simulink model "FYPPP"  (R2021b)
settings: Solver=VariableStepAuto  StartTime=0.0  StopTime=7200  MaxStep=10  RelTol=1e-3  EnableMultiTasking=on
PreLoadFcn:
  | ssc_lithium_cell_1RC_ini
undefined symbols (not defined in the file): Battery, C1, Capacity, DiscIntNeverNeededParam, Em, Ion, Lithium, Qe_init, R0, R1
libraries: fl_lib x50, nesl_utility x17, LiBatteryElements_lib x12, fl_ps_legacy_lib x9, spsBatteryLib x4, spsSeriesRLCBranchLib x4, spsIGBTLib x3, ee_lib x2, spsIdealSwitchLib x2, spsBreakerLib x2, spspowerguiLib x2, spsDCVoltageSourceLib x1
(part 1 of 2)
CloseFcn:
  | try,close(h1_ssc_lithium_battery_with_fault),end
  | clear h1_ssc_lithium_battery_with_fault
  | 
  | clear simlog_ssc_lithium_battery_with_fault
Description:
  | Lithium-Ion Battery Pack With Fault
  | 
  | Copyright 2008-2017 The MathWorks, Inc.
settings Model: Creator=MathWorks  LastModifiedBy=91875
settings SolverCC: AlgebraicLoopSolver=TrustRegion
settings DataIOCC: LimitDataPoints=on  SaveFormat=Array  ReturnWorkspaceOutputs=off
settings OptimizationCC: LifeSpan=inf
settings DebuggingCC: AllowSymbolicDim=off  SFUnexpectedBacktrackingDiag=warning  SFNoUnconditionalDefaultTransitionDiag=warning  SFExecutionAtInitializationDiag=none  SFMachineParentedDataDiag=warning  ArithmeticOperatorsInVariantConditions=warning
settings HardwareCC: ProdBitPerPointer=32  ProdBitPerSizeT=32  ProdBitPerPtrDiffT=32  ProdLargestAtomicFloat=None  ProdIntDivRoundTo=Undefined  ProdEndianess=Unspecified  ProdWordSize=32  ProdHWDeviceType=32-bit Generic
settings ModelReferenceCC: PropagateSignalLabelsOutOfModel=off
settings SFSimCC: SimUseLocalCustomCode=off  CustomCodeUndefinedFunction=UseInterfaceOnly
settings RTWCC: RTWUseLocalCustomCode=off
settings CodeAppCC: StateflowObjectComments=on
settings GRTTargetCC: TargetLangStandard=C89/C90 (ANSI)
settings ConfigComp: CovMetricSettings=dw  CovSaveCumulativeToWorkspaceVar=on  CovSaveSingleToWorkspaceVar=on  CovExternalEMLEnable=off
settings SimscapeCC: SimscapeNormalizeSystem=off  SimscapeLogType=all  SimscapeLogSimulationStatistics=on  SimscapeLogName=simlog_ssc_lithium_battery_with_fault  SimscapeLogDataHistory=10000

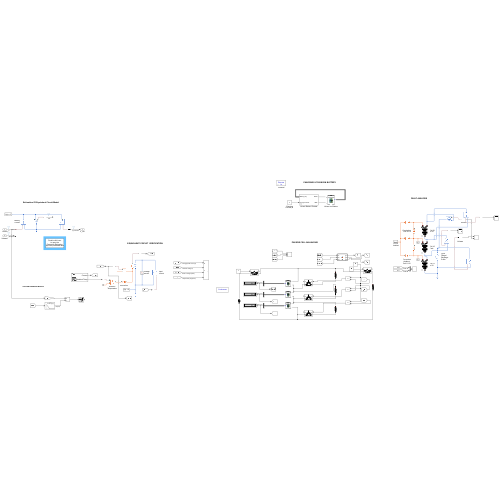
[thumbnail: Simulink's stored preview of the top-level diagram]
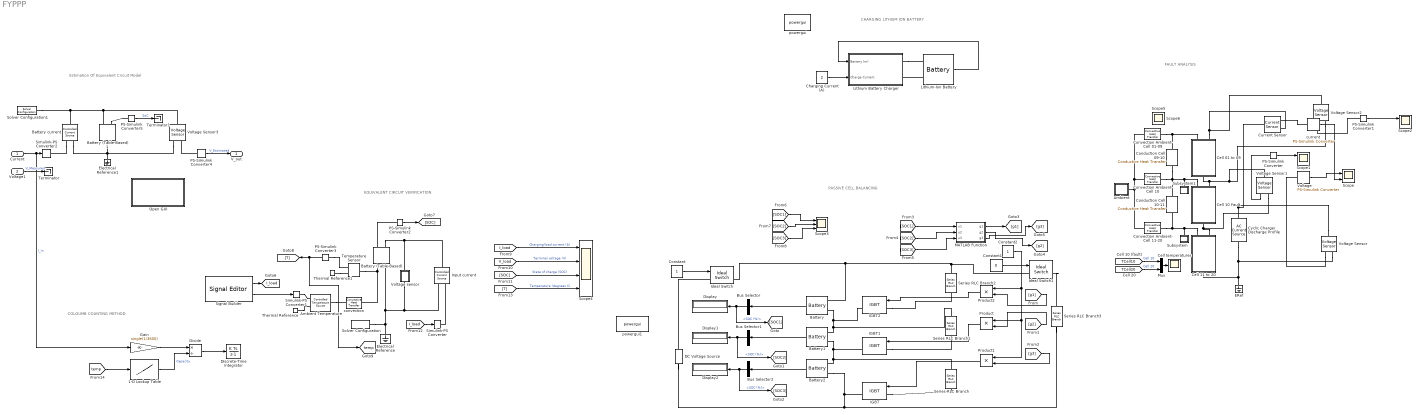
== system FYPPP ==
  note: COLOUMB COUNTING METHOD
  note: Estimation Of Equivalent Circuit Model
  note: EQUIVALENT CIRCUIT VERIFICATION
  note: PASSIVE CELL BALANCING
  note: CHARGING LITHIUM ION BATTERY
  note: FAULT ANALYSIS
  Current : Inport
  Voltage1 : Inport  Port=2
  1-D Lookup Table : Lookup_n-D  NumberOfTableDimensions=1  BreakpointsForDimension1=single(Battery(1).Temperature_LUT)  Table=single(Battery(1).Capacity_LUT)  InternalRulePriority=Speed  RndMeth=Simplest  InputSameDT=on
  Ambient : Subsystem
  Ambient Temperature : fl_lib/Thermal/Thermal Sources/Controlled Temperature Source
  Battery : spsBatteryLib/Battery  BatType=Lithium-Ion  ShowTempParam=off  ThermalPreset=no  ShowAgeParam=off  NomV=3.7  NomQ=5.4  SOC=32  Batt_Tr=30  PresetModel=on  MaxQ=5.4  MinV=2.775  FullV=4.3068  Dis_rate=2.3478  R=0.0068519  Normal_OP=4.8835  expZone="[3.9974      0.2653]"  current=[6.5 13 32.5]  Units=Time  Tci=20  NomT=20  T2=-30  MaxQ2=4.8  FullV2=7.1  Normal_OP2=5.655  expZone2="[6.58           1]"  Rca=0.6  ti=2000  Dp=0  Neq0=0  Tsim=1e6  Ta1=25  Qeol=5.4*0.9  Reol=0.013333*1.2  Char_age=[2.3478, 3]  Dis_age=[2.3478, 10]  N1=1500  N2=10500  N3=1000  N4=1400  Ta2=45  N5=950
  Battery (Table-Based) : ee_lib/Sources/Battery (Table-Based)  SOC_vec=Battery.SOC_LUT  T_dependence=ee.enum.temperature_dependence.yes  prm_dir=ee.enum.battery.prm_dir.noCurrentDirectionality  T_vec=Battery.Temperature_LUT K  V0_mat=Battery.Em_LUT V  V0_vec=[3.1, 3.27, 3.31, 3.5] V  R0_mat=Battery.R0_LUT Ohm  R0_vec=[.015, .017, .012, .013] Ohm  R0_dis_mat=[.03, .015, .002; .04, .017, .008; .039, .012, .006; .027, .013, .021] Ohm  R0_dis_vec=[.015, .017, .012, .013] Ohm  R0_ch_mat=[.03, .015, .002; .04, .017, .008; .039, .012, .006; .027, .013, .021] Ohm  R0_ch_vec=[.015, .017, .012, .013] Ohm  AH_vec=Battery.Capacity_LUT hr*A  AH=4.1 hr*A  prm_leak=1  Rleak_vec=[8000, 7000, 6000] Ohm  Rleak=7e3 Ohm  extrapolation_option=ee.enum.extrapolation.linear  prm_dyn=2  R1_mat=Battery.R1_LUT Ohm  R1_vec=[.076, .022, .007, .043] Ohm  tau1_mat=Battery.R1_LUT.*Battery.C1_LUT s  tau1_vec=[148, 110, 27, 22] s  R2_mat=[.014, .382, .407; .028, .006, .007; .014, .007, .006; .333, .956, .912] Ohm  R2_vec=[.382, .006, .007, .956] Ohm  tau2_mat=[1, 44, 5644; 11, 24, 506; 2, 14, 330; 3310, 13419, 30216] s  tau2_vec=[44, 24, 14, 13419] s  R3_mat=[.014, .382, .407; .028, .006, .007; .014, .007, .006; .333, .956, .912] Ohm  R3_vec=[.382, .006, .007, .956] Ohm  tau3_mat=[1, 44, 5644; 11, 24, 506; 2, 14, 330; 3310, 13419, 30216] s  tau3_vec=[44, 24, 14, 13419] s  R4_mat=[.014, .382, .407; .028, .006, .007; .014, .007, .006; .333, .956, .912] Ohm  R4_vec=[.382, .006, .007, .956] Ohm  tau4_mat=[1, 44, 5644; 11, 24, 506; 2, 14, 330; 3310, 13419, 30216] s  tau4_vec=[44, 24, 14, 13419] s  R5_mat=[.014, .382, .407; .028, .006, .007; .014, .007, .006; .333, .956, .912] Ohm  R5_vec=[.382, .006, .007, .956] Ohm  tau5_mat=[1, 44, 5644; 11, 24, 506; 2, 14, 330; 3310, 13419, 30216] s  tau5_vec=[44, 24, 14, 13419] s  prm_fade=ee.enum.battery.prm_fade.equations  N0=100  dV0=0  dR0=0  dAH=0  dRleak=0  dR1=0  dR2=0  dR3=0  dR4=0  dR5=0  N0vec=[100, 200, 300]  Tfadevec=[298.15, 323.15] K  dV0vec=[0, 0, 0]  dR0vec=[0, 0, 0]  dAHvec=[0, 0, 0]  dRleakvec=[0, 0, 0]  dR1vec=[0, 0, 0]  dR2vec=[0, 0, 0]  dR3vec=[0, 0, 0]  dR4vec=[0, 0, 0]  dR5vec=[0, 0, 0]  dV0mat=[0, 0; 0, 0; 0, 0]  dR0mat=[0, 0; 0, 0; 0, 0]  dAHmat=[0, 0; 0, 0; 0, 0]  dRleakmat=[0, 0; 0, 0; 0, 0]  dR1mat=[0, 0; 0, 0; 0, 0]  dR2mat=[0, 0; 0, 0; 0, 0]  dR3mat=[0, 0; 0, 0; 0, 0]  dR4mat=[0, 0; 0, 0; 0, 0]  dR5mat=[0, 0; 0, 0; 0, 0]  prm_age=ee.enum.battery.prm_age.disabled  prm_age_OCV=ee.enum.battery.prm_age_OCV.OCV  OCV_age=0.9  SOC_age=0.6  storage_dt_age_vec=[0] d  storage_T_age_vec=[273] K  OCV_scaling_age=2.2134e6  OCV_offset_age=1.632e6  temp_exp_age=0.515833569 V  t_exp_age=0.75  T_age_vec=[273.15, 298.15, 323.15] K  dt_age_vec=[90, 180, 270, 360] d  dR0_age_vec=[0, 0, 0]  t_meas_dR0_age=100 d  dR0_age_mat=[0, 0, 0; 0, 0, 0; 0, 0, 0; 0, 0, 0]  temperature=Battery.T_init K  i_specify=off  i_priority=None  i=0 A  i_nominal_specify=off  i_nominal_unit=A  i_nominal_value=1  v_specify=off  v_priority=None  v=0 V  v_nominal_specify=off  v_nominal_unit=V  v_nominal_value=1  stateOfCharge_specify=on  stateOfCharge_priority=High  stateOfCharge=(Battery.Capacity_LUT(2) - Battery.Qe_init)/Battery.Capacity_LUT(2)  stateOfCharge_nominal_specify=off  stateOfCharge_nominal_unit=1  stateOfCharge_nominal_value=1  num_cycles_specify=off  num_cycles_priority=High  num_cycles=0  num_cycles_nominal_specify=off  num_cycles_nominal_unit=1  num_cycles_nominal_value=1  thermal_mass=Battery.cell_Cp_heat*Battery.cell_mass J/K  temperature_specify=on  temperature_priority=High  temperature_nominal_specify=off  temperature_nominal_unit=K  temperature_nominal_value=1
      settings: SourceProductBaseCode=PS  InternalSimscapePortConfiguration="{\"Bottom\":[],\"Left\":[{\"id\":\"p\",\"label\":\"+\",\"type\":\"foundation.electrical.electrical\"},{\"id\":\"soc\",\"label\":\"SOC\",\"type\":\"output\"}],\"Right\":[{\"id\":\"n\",\"label\":\"-\",\"type\":\"foundation.electrical.electrical\"},{\"id\":\"H\",\"label\":\"H\",\"type\":\"foundation.thermal.thermal\"}],\"Top\":[]}"
  Battery (Table-Based)1 : ee_lib/Sources/Battery (Table-Based)  SOC_vec=SOC_LUT  T_dependence=ee.enum.temperature_dependence.no  prm_dir=ee.enum.battery.prm_dir.noCurrentDirectionality  T_vec=[273.15, 298.15] K  V0_mat=[Em, Em] V  V0_vec=Em V  R0_mat=[R0, R0] Ohm  R0_vec=R0 Ohm  R0_dis_mat=[.03, .015, .002; .04, .017, .008; .039, .012, .006; .027, .013, .021] Ohm  R0_dis_vec=[.015, .017, .012, .013] Ohm  R0_ch_mat=[.03, .015, .002; .04, .017, .008; .039, .012, .006; .027, .013, .021] Ohm  R0_ch_vec=[.015, .017, .012, .013] Ohm  AH_vec=[Capacity, Capacity] hr*A  AH=Capacity hr*A  prm_leak=ee.enum.battery.prm_leak.disabled  Rleak_vec=[8000, 7000, 6000] Ohm  Rleak=7e3 Ohm  extrapolation_option=ee.enum.extrapolation.linear  prm_dyn=ee.enum.battery.prm_dyn.rc1  R1_mat=[R1, R1] Ohm  R1_vec=R1 Ohm  tau1_mat=[R1.*C1, R1.*C1] s  tau1_vec=R1.*C1 s  R2_mat=[.014, .382, .407; .028, .006, .007; .014, .007, .006; .333, .956, .912] Ohm  R2_vec=[.382, .006, .007, .956] Ohm  tau2_mat=[1, 44, 5644; 11, 24, 506; 2, 14, 330; 3310, 13419, 30216] s  tau2_vec=[44, 24, 14, 13419] s  R3_mat=[.014, .382, .407; .028, .006, .007; .014, .007, .006; .333, .956, .912] Ohm  R3_vec=[.382, .006, .007, .956] Ohm  tau3_mat=[1, 44, 5644; 11, 24, 506; 2, 14, 330; 3310, 13419, 30216] s  tau3_vec=[44, 24, 14, 13419] s  R4_mat=[.014, .382, .407; .028, .006, .007; .014, .007, .006; .333, .956, .912] Ohm  R4_vec=[.382, .006, .007, .956] Ohm  tau4_mat=[1, 44, 5644; 11, 24, 506; 2, 14, 330; 3310, 13419, 30216] s  tau4_vec=[44, 24, 14, 13419] s  R5_mat=[.014, .382, .407; .028, .006, .007; .014, .007, .006; .333, .956, .912] Ohm  R5_vec=[.382, .006, .007, .956] Ohm  tau5_mat=[1, 44, 5644; 11, 24, 506; 2, 14, 330; 3310, 13419, 30216] s  tau5_vec=[44, 24, 14, 13419] s  prm_fade=ee.enum.battery.prm_fade.equations  N0=100  dV0=0  dR0=0  dAH=0  dRleak=0  dR1=0  dR2=0  dR3=0  dR4=0  dR5=0  N0vec=[100, 200, 300]  Tfadevec=[298.15, 323.15] K  dV0vec=[0, 0, 0]  dR0vec=[0, 0, 0]  dAHvec=[0, 0, 0]  dRleakvec=[0, 0, 0]  dR1vec=[0, 0, 0]  dR2vec=[0, 0, 0]  dR3vec=[0, 0, 0]  dR4vec=[0, 0, 0]  dR5vec=[0, 0, 0]  dV0mat=[0, 0; 0, 0; 0, 0]  dR0mat=[0, 0; 0, 0; 0, 0]  dAHmat=[0, 0; 0, 0; 0, 0]  dRleakmat=[0, 0; 0, 0; 0, 0]  dR1mat=[0, 0; 0, 0; 0, 0]  dR2mat=[0, 0; 0, 0; 0, 0]  dR3mat=[0, 0; 0, 0; 0, 0]  dR4mat=[0, 0; 0, 0; 0, 0]  dR5mat=[0, 0; 0, 0; 0, 0]  prm_age=ee.enum.battery.prm_age.disabled  prm_age_OCV=ee.enum.battery.prm_age_OCV.OCV  OCV_age=0.9  SOC_age=0.6  storage_dt_age_vec=[0] d  storage_T_age_vec=[273] K  OCV_scaling_age=2.2134e6  OCV_offset_age=1.632e6  temp_exp_age=0.515833569 V  t_exp_age=0.75  T_age_vec=[273.15, 298.15, 323.15] K  dt_age_vec=[90, 180, 270, 360] d  dR0_age_vec=[0, 0, 0]  t_meas_dR0_age=100 d  dR0_age_mat=[0, 0, 0; 0, 0, 0; 0, 0, 0; 0, 0, 0]  temperature=298.15 K  i_specify=off  i_priority=None  i=0 A  i_nominal_specify=off  i_nominal_unit=A  i_nominal_value=1  v_specify=off  v_priority=None  v=0 V  v_nominal_specify=off  v_nominal_unit=V  v_nominal_value=1  stateOfCharge_specify=off  stateOfCharge_priority=High  stateOfCharge=1  stateOfCharge_nominal_specify=off  stateOfCharge_nominal_unit=1  stateOfCharge_nominal_value=1  num_cycles_specify=off  num_cycles_priority=High  num_cycles=0  num_cycles_nominal_specify=off  num_cycles_nominal_unit=1  num_cycles_nominal_value=1  thermal_mass=30000 J/K  temperature_specify=off  temperature_priority=High  temperature_nominal_specify=off  temperature_nominal_unit=K  temperature_nominal_value=1
      settings: SourceProductBaseCode=PS  InternalSimscapePortConfiguration="{\"Bottom\":[],\"Left\":[{\"id\":\"p\",\"label\":\"+\",\"type\":\"foundation.electrical.electrical\"},{\"id\":\"soc\",\"label\":\"SOC\",\"type\":\"output\"}],\"Right\":[{\"id\":\"n\",\"label\":\"-\",\"type\":\"foundation.electrical.electrical\"}],\"Top\":[]}"
  Battery current : fl_lib/Electrical/Electrical Sources/Controlled Current Source
  Battery1 : spsBatteryLib/Battery  BatType=Lithium-Ion  ShowTempParam=off  ThermalPreset=no  ShowAgeParam=off  NomV=3.7  NomQ=5.4  SOC=28  Batt_Tr=30  PresetModel=on  MaxQ=5.4  MinV=2.775  FullV=4.3068  Dis_rate=2.3478  R=0.0068519  Normal_OP=4.8835  expZone="[3.9974      0.2653]"  current=[6.5 13 32.5]  Units=Time  Tci=20  NomT=20  T2=-30  MaxQ2=4.8  FullV2=7.1  Normal_OP2=5.655  expZone2="[6.58           1]"  Rca=0.6  ti=2000  Dp=0  Neq0=0  Tsim=1e6  Ta1=25  Qeol=5.4*0.9  Reol=0.013333*1.2  Char_age=[2.3478, 3]  Dis_age=[2.3478, 10]  N1=1500  N2=10500  N3=1000  N4=1400  Ta2=45  N5=950
  Battery2 : spsBatteryLib/Battery  BatType=Lithium-Ion  ShowTempParam=off  ThermalPreset=no  ShowAgeParam=off  NomV=3.7  NomQ=5.4  SOC=26  Batt_Tr=30  PresetModel=on  MaxQ=5.4  MinV=2.775  FullV=4.3068  Dis_rate=2.3478  R=0.0068519  Normal_OP=4.8835  expZone="[3.9974      0.2653]"  current=[6.5 13 32.5]  Units=Time  Tci=20  NomT=20  T2=-30  MaxQ2=4.8  FullV2=7.1  Normal_OP2=5.655  expZone2="[6.58           1]"  Rca=0.6  ti=2000  Dp=0  Neq0=0  Tsim=1e6  Ta1=25  Qeol=5.4*0.9  Reol=0.013333*1.2  Char_age=[2.3478, 3]  Dis_age=[2.3478, 10]  N1=1500  N2=10500  N3=1000  N4=1400  Ta2=45  N5=950
  Bus Selector : BusSelector  OutputSignals=SOC (%)
  Bus Selector1 : BusSelector  OutputSignals=SOC (%)
  Bus Selector2 : BusSelector  OutputSignals=SOC (%)
  Cell temperatures : Scope
  Cell 01 to 09 : Subsystem  Tag=PublishSubsystem  mask(Lithium cell (one RC-branch equivalent circuit)){Ncells=9, Qe_init=Qe_init, T_init=Battery.T_init, Capacity_LUT=Battery.Capacity_LUT, Em_LUT=Battery.Em_LUT, R0_LUT=Battery.R0_LUT, R1_LUT=Battery.R1_LUT, C1_LUT=Battery.C1_LUT, cell_mass=Battery.cell_mass, cell_Cp_heat=Battery.cell_Cp_heat, SOC_LUT=Battery.SOC_LUT, Temperature_LUT=Battery.Temperature_LUT}
      mask prompts: Ncells "Number of series-connected cells"; Qe_init "Initial cell charge deficit (A*hr)"; T_init "Initial cell temperature (K)"; Capacity_LUT "Capacity (A*hr, 1xN table)"; Em_LUT "Em open-circuit voltage, Em (volts, MxN table)"; R0_LUT "R0 terminal resistance (ohms, MxN table)"; R1_LUT "R1 cell resistance (ohms, MxN table)"; C1_LUT "C1 capacitance (farads, MxN table)"; cell_mass "Cell mass (kg)"; cell_Cp_heat "Cell specific heat (J/kg/K)"; SOC_LUT "SOC table breakpoints (Mx1 array)"; Temperature_LUT "Temperature table breakpoints (K, 1xN array)"
      mask DialogControl ParameterTabVar0 Prompt: Main
      mask DialogControl ParameterTabVar01 Prompt: Electrical (per cell)
      mask DialogControl ParameterTabVar012 Prompt: Thermal (per cell)
      mask DialogControl ParameterTabVar0123 Prompt: Table Breakpoints
      mask Display:
      | % Battery icon
      | plot([2.5 1.3],[0 0])
      | plot([-0.6 -1.6 -1.6 -2.5],[0 0 -0.8 -0.8])
      | patch([1 1 -1 -1]*0.15+1.3,[-1 1 1 -1]*0.4,[0;0;0]);
      | patch([1 1 -1 -1]*0.15+0.0,[-1 1 1 -1]*0.4,[0;0;0]);
      | patch([1 1 -1 -1]*0.15+0.7,[-1 1 1 -1]*0.8,[0;0;0]);
      | patch([1 1 -1 -1]*0.15-0.6,[-1 1 1 -1]*0.8,[0;0;0]);
      | % Thermal port
      | plot([-1.6,-1.3],[1.2,1.2])
      | plot([-1.6,-1.3],[0.5,0.5])
      | plot([-1.6,-2.5],[0.8,0.8])
      | plot(0.2*sin(0:2*pi/50:2*pi)-1.6,0.35*cos(0:2*pi/50:2*pi)+0.85)
      | plot(0.2*sin(0:2*pi/50:pi)-1.3,0.35*cos(0:2*pi/50:pi)+0.85)
      | 
      | % Plot points to set plot range
      | color('white');plot(2.5,1.5);plot(-2.5,-1.5)
      | 
      | color('red')
      | port_label('LConn',1,'H')
      | port_label('LConn',2,'+')
      | port_label('RConn',1,'-')
  Cell 10 Fault : Subsystem  mask(Lithium cell (one RC-branch equivalent circuit)){Ncells=1, Qe_init=Qe_init, T_init=Battery.T_init, Capacity_LUT=Battery.Capacity_LUT*0.9, Em_LUT=Battery.Em_LUT*0.9, R0_LUT=Battery.R0_LUT*5, R1_LUT=Battery.R1_LUT*5, C1_LUT=Battery.C1_LUT, cell_mass=Battery.cell_mass, cell_Cp_heat=Battery.cell_Cp_heat, SOC_LUT=Battery.SOC_LUT, Temperature_LUT=Battery.Temperature_LUT}
      mask prompts: Ncells "Number of series-connected cells"; Qe_init "Initial cell charge deficit (A*hr)"; T_init "Initial cell temperature (K)"; Capacity_LUT "Capacity (A*hr, 1xN table)"; Em_LUT "Em open-circuit voltage, Em (volts, MxN table)"; R0_LUT "R0 terminal resistance (ohms, MxN table)"; R1_LUT "R1 cell resistance (ohms, MxN table)"; C1_LUT "C1 capacitance (farads, MxN table)"; cell_mass "Cell mass (kg)"; cell_Cp_heat "Cell specific heat (J/kg/K)"; SOC_LUT "SOC table breakpoints (Mx1 array)"; Temperature_LUT "Temperature table breakpoints (K, 1xN array)"
      mask DialogControl ParameterTabVar0 Prompt: Main
      mask DialogControl ParameterTabVar01 Prompt: Electrical (per cell)
      mask DialogControl ParameterTabVar012 Prompt: Thermal (per cell)
      mask DialogControl ParameterTabVar0123 Prompt: Table Breakpoints
      mask Display:
      | % Battery icon
      | plot([2.5 1.3],[0 0])
      | plot([-0.6 -1.6 -1.6 -2.5],[0 0 -0.8 -0.8])
      | patch([1 1 -1 -1]*0.15+1.3,[-1 1 1 -1]*0.4,[0;0;0]);
      | patch([1 1 -1 -1]*0.15+0.0,[-1 1 1 -1]*0.4,[0;0;0]);
      | patch([1 1 -1 -1]*0.15+0.7,[-1 1 1 -1]*0.8,[0;0;0]);
      | patch([1 1 -1 -1]*0.15-0.6,[-1 1 1 -1]*0.8,[0;0;0]);
      | % Thermal port
      | plot([-1.6,-1.3],[1.2,1.2])
      | plot([-1.6,-1.3],[0.5,0.5])
      | plot([-1.6,-2.5],[0.8,0.8])
      | plot(0.2*sin(0:2*pi/50:2*pi)-1.6,0.35*cos(0:2*pi/50:2*pi)+0.85)
      | plot(0.2*sin(0:2*pi/50:pi)-1.3,0.35*cos(0:2*pi/50:pi)+0.85)
      | 
      | % Plot points to set plot range
      | color('white');plot(2.5,1.5);plot(-2.5,-1.5)
      | 
      | color('red')
      | port_label('LConn',1,'H')
      | port_label('LConn',2,'+')
      | port_label('RConn',1,'-')
  Cell 11 to 20 : Subsystem  mask(Lithium cell (one RC-branch equivalent circuit)){Ncells=10, Qe_init=Qe_init, T_init=Battery.T_init, Capacity_LUT=Battery.Capacity_LUT, Em_LUT=Battery.Em_LUT, R0_LUT=Battery.R0_LUT, R1_LUT=Battery.R1_LUT, C1_LUT=Battery.C1_LUT, cell_mass=Battery.cell_mass, cell_Cp_heat=Battery.cell_Cp_heat, SOC_LUT=Battery.SOC_LUT, Temperature_LUT=Battery.Temperature_LUT}
      mask prompts: Ncells "Number of series-connected cells"; Qe_init "Initial cell charge deficit (A*hr)"; T_init "Initial cell temperature (K)"; Capacity_LUT "Capacity (A*hr, 1xN table)"; Em_LUT "Em open-circuit voltage, Em (volts, MxN table)"; R0_LUT "R0 terminal resistance (ohms, MxN table)"; R1_LUT "R1 cell resistance (ohms, MxN table)"; C1_LUT "C1 capacitance (farads, MxN table)"; cell_mass "Cell mass (kg)"; cell_Cp_heat "Cell specific heat (J/kg/K)"; SOC_LUT "SOC table breakpoints (Mx1 array)"; Temperature_LUT "Temperature table breakpoints (K, 1xN array)"
      mask DialogControl ParameterTabVar0 Prompt: Main
      mask DialogControl ParameterTabVar01 Prompt: Electrical (per cell)
      mask DialogControl ParameterTabVar012 Prompt: Thermal (per cell)
      mask DialogControl ParameterTabVar0123 Prompt: Table Breakpoints
      mask Display:
      | % Battery icon
      | plot([2.5 1.3],[0 0])
      | plot([-0.6 -1.6 -1.6 -2.5],[0 0 -0.8 -0.8])
      | patch([1 1 -1 -1]*0.15+1.3,[-1 1 1 -1]*0.4,[0;0;0]);
      | patch([1 1 -1 -1]*0.15+0.0,[-1 1 1 -1]*0.4,[0;0;0]);
      | patch([1 1 -1 -1]*0.15+0.7,[-1 1 1 -1]*0.8,[0;0;0]);
      | patch([1 1 -1 -1]*0.15-0.6,[-1 1 1 -1]*0.8,[0;0;0]);
      | % Thermal port
      | plot([-1.6,-1.3],[1.2,1.2])
      | plot([-1.6,-1.3],[0.5,0.5])
      | plot([-1.6,-2.5],[0.8,0.8])
      | plot(0.2*sin(0:2*pi/50:2*pi)-1.6,0.35*cos(0:2*pi/50:2*pi)+0.85)
      | plot(0.2*sin(0:2*pi/50:pi)-1.3,0.35*cos(0:2*pi/50:pi)+0.85)
      | 
      | % Plot points to set plot range
      | color('white');plot(2.5,1.5);plot(-2.5,-1.5)
      | 
      | color('red')
      | port_label('LConn',1,'H')
      | port_label('LConn',2,'+')
      | port_label('RConn',1,'-')
  Charging Current (A) : Constant  Value=2
  Conduction Cell 09-10 : fl_lib/Thermal/Thermal Elements/Conductive Heat Transfer  area=1e-3 m^2  thickness=0.1 m  th_cond=200 W/(m*K)  T_specify=off  T_priority=High  T=0 K  T_nominal_specify=off  T_nominal_unit=K  T_nominal_value=1  Q_specify=off  Q_priority=High  Q=0 J/s  Q_nominal_specify=off  Q_nominal_unit=J/s  Q_nominal_value=1
  "Conduction Cell 10-11 " : fl_lib/Thermal/Thermal Elements/Conductive Heat Transfer  area=1e-3 m^2  thickness=0.1 m  th_cond=200 W/(m*K)  T_specify=off  T_priority=High  T=0 K  T_nominal_specify=off  T_nominal_unit=K  T_nominal_value=1  Q_specify=off  Q_priority=High  Q=0 J/s  Q_nominal_specify=off  Q_nominal_unit=J/s  Q_nominal_value=1
  Constant : Constant
  Constant1 : Constant  Value=0
  Constant2 : Constant
  Convection Ambient- Cell 01-09 : fl_lib/Thermal/Thermal Elements/Convective Heat Transfer  area=Battery.cell_area*9 m^2  heat_tr_coeff=Battery.h_conv W/(m^2*K)  T_specify=off  T_priority=High  T=0 K  T_nominal_specify=off  T_nominal_unit=K  T_nominal_value=1  Q_specify=off  Q_priority=High  Q=0 J/s  Q_nominal_specify=off  Q_nominal_unit=J/s  Q_nominal_value=1
  Convection Ambient- Cell 10 : fl_lib/Thermal/Thermal Elements/Convective Heat Transfer  area=Battery.cell_area m^2  heat_tr_coeff=Battery.h_conv W/(m^2*K)  T_specify=off  T_priority=High  T=0 K  T_nominal_specify=off  T_nominal_unit=K  T_nominal_value=1  Q_specify=off  Q_priority=High  Q=0 J/s  Q_nominal_specify=off  Q_nominal_unit=J/s  Q_nominal_value=1
  Convection Ambient- Cell 11-20 : fl_lib/Thermal/Thermal Elements/Convective Heat Transfer  area=Battery.cell_area*10 m^2  heat_tr_coeff=Battery.h_conv W/(m^2*K)  T_specify=off  T_priority=High  T=0 K  T_nominal_specify=off  T_nominal_unit=K  T_nominal_value=1  Q_specify=off  Q_priority=High  Q=0 J/s  Q_nominal_specify=off  Q_nominal_unit=J/s  Q_nominal_value=1
  Current Sensor : fl_lib/Electrical/Electrical Sensors/Current Sensor
  Cyclic Charge/ Discharge Profile : fl_lib/Electrical/Electrical Sources/AC Current Source  amp=50 A  shift=0 deg  frequency=1/1000 Hz  omega=0 rad/s
      settings: SourceProductBaseCode=SS  InternalSimscapePortConfiguration="{\"Bottom\":[],\"Left\":[{\"id\":\"p\",\"label\":\"\",\"type\":\"foundation.electrical.electrical\"}],\"Right\":[{\"id\":\"n\",\"label\":\"\",\"type\":\"foundation.electrical.electrical\"}],\"Top\":[]}"
  DC Voltage Source : spsDCVoltageSourceLib/DC Voltage Source  Amplitude=12  Measurements=None
  Discrete-Time Integrator : DiscreteIntegrator  InitialCondition=single(0+0.05)  SampleTime=-1  LimitOutput=on  UpperSaturationLimit=1  LowerSaturationLimit=0  ICPrevOutput=DiscIntNeverNeededParam  ICPrevScaledInput=DiscIntNeverNeededParam
  Display : Display
  Display1 : Display
  Display2 : Display
  Divide : Product  Inputs=*/
  "ERef " : fl_lib/Electrical/Electrical Elements/Electrical Reference
  Electrical Reference : fl_lib/Electrical/Electrical Elements/Electrical Reference
  Electrical Reference1 : fl_lib/Electrical/Electrical Elements/Electrical Reference
  Gain : Gain  Gain=single(1/3600)
  IGBT : spsIGBTLib/IGBT  Ron=0.001  Lon=0  Vf=1  Tf=1e-6  Tt=2e-6  IC=0  Rs=1e5  Cs=inf  Measurements=on
  IGBT1 : spsIGBTLib/IGBT  Ron=0.001  Lon=0  Vf=1  Tf=1e-6  Tt=2e-6  IC=0  Rs=1e5  Cs=inf  Measurements=on
  IGBT2 : spsIGBTLib/IGBT  Ron=0.001  Lon=0  Vf=1  Tf=1e-6  Tt=2e-6  IC=0  Rs=1e5  Cs=inf  Measurements=on
  Ideal Switch : spsIdealSwitchLib/Ideal Switch  Ron=0.001  Lon=0  IC=0  Rs=1e5  Cs=inf  Measurements=on
  Ideal Switch1 : spsIdealSwitchLib/Ideal Switch  Ron=0.001  Lon=0  IC=0  Rs=1e5  Cs=inf  Measurements=on
  Input current : fl_lib/Electrical/Electrical Sources/Controlled Current Source
  Lithium Battery Charger : Subsystem  mask(Lithium Battery Charger){CV=4.2}
      mask prompts: CV "Saturation Charge Constant Voltage (V)"
      mask help:
      | Lithium Battery Charger Block Developed By Rodney Tan (PhD)
      | Version 1.00 (Aug 2019)
      |
      | This charger charge Lithium-Ion battery in two stages
      | This charger takes in charge current (A) from the input in (CC) Constant Current charging stage and switch to Saturation Charge (CV) Constant Voltage charging stage when the battery reaches the set constant voltage.
  Lithium-Ion Battery : spsBatteryLib/Battery  BatType=Lithium-Ion  ShowTempParam=off  ThermalPreset=no  ShowAgeParam=off  NomV=3.7  NomQ=3.2  SOC=50  Batt_Tr=30  PresetModel=on  MaxQ=3.2  MinV=2.775  FullV=4.3068  Dis_rate=1.3913  R=0.011562  Normal_OP=2.8939  expZone="[3.9974     0.15722]"  current=[1.2 0.6 0.3]  Units=Time  Tci=20  NomT=25  T2=0  MaxQ2=2.208  FullV2=3.45  Normal_OP2=2.8  expZone2="[3.22        0.23]"  Rca=0.6  ti=1000  Dp=0  Neq0=0  Tsim=1e6  Ta1=25  Qeol=5.4*0.9  Reol=0.013333*1.2  Char_age=[2.3478, 3]  Dis_age=[2.3478, 10]  N1=1500  N2=10500  N3=1000  N4=1400  Ta2=45  N5=950
  MATLAB Function : MATLAB Function  TreatAsAtomicUnit=on
  Mux : Mux  Inputs=2
  Open GUI : Subsystem
      settings: OpenFcn=|
      | % speload('ssc_lithium_cell_SDO_Project', 'Project - ssc_lithium_cell_1RC_estim', 'One Temp Estim');
      | spetool('ssc_lithium_cell_1RC_estim_spesession')
      mask Display: disp('Double click here\nto open the\nParameter Estimation\nApp with preloaded data')
  PS-Simulink Converter : nesl_utility/PS-Simulink Converter  PhysicalDomain=network_engine_domain  SubClassName=ps_output  LeftPortType=input  RightPortType=output  PseudoPeriodic=off  Frequencies=[]  Unit=inherit  AffineConversion=off
      settings: SourceProductBaseCode=PW,SS
  PS-Simulink Converter1 : nesl_utility/PS-Simulink Converter  PhysicalDomain=network_engine_domain  SubClassName=ps_output  LeftPortType=input  RightPortType=output  PseudoPeriodic=off  Frequencies=[]  Unit=inherit  AffineConversion=off
      settings: SourceProductBaseCode=PW,SS
  PS-Simulink Converter2 : nesl_utility/PS-Simulink Converter  PhysicalDomain=network_engine_domain  SubClassName=ps_output  LeftPortType=input  RightPortType=output  PseudoPeriodic=off  Frequencies=[]  Unit=1  AffineConversion=off
      settings: SourceProductBaseCode=PW,SS
  PS-Simulink Converter3 : nesl_utility/PS-Simulink Converter  PhysicalDomain=network_engine_domain  SubClassName=ps_output  LeftPortType=input  RightPortType=output  PseudoPeriodic=off  Frequencies=[]  Unit=K  AffineConversion=off
      settings: SourceProductBaseCode=PW,SS
  PS-Simulink Converter4 : nesl_utility/PS-Simulink Converter  PhysicalDomain=network_engine_domain  SubClassName=ps_output  LeftPortType=input  RightPortType=output  PseudoPeriodic=off  Frequencies=[]  Unit=V  AffineConversion=off
      settings: SourceProductBaseCode=PW,SS
  PS-Simulink Converter5 : nesl_utility/PS-Simulink Converter  PhysicalDomain=network_engine_domain  SubClassName=ps_output  LeftPortType=input  RightPortType=output  PseudoPeriodic=off  Frequencies=[]  Unit=1  AffineConversion=off
      settings: SourceProductBaseCode=PW,SS
  Product : Product
  Product1 : Product
  Product2 : Product
  Scope : Scope  NumInputPorts=2
  Scope1 : Scope  NumInputPorts=2
  Scope2 : Scope  NumInputPorts=2
  Scope3 : Scope  NumInputPorts=3
  Scope4 : Scope  NumInputPorts=4
  Series RLC Branch{,1..3} (4 alike) : spsSeriesRLCBranchLib/Series RLC Branch  LConnTagsString=__new0  RConnTagsString=__new0  BranchType=R  Resistance=1  Inductance=1e-3  SetiL0=off  InitialCurrent=0  Capacitance=1e-6  Setx0=on  InitialVoltage=0  Measurements=None
  Signal Builder : SignalEditorBlockLib/Signal Editor  FileName=C:\Users\91875\Downloads\BatteryManagementSystem\Battery_System_R2020a\SignalBuilder.mat  ActiveScenario=Pulse  ActiveSignal=Ambient Temp  IsBus=off  OutputBusObjectStr=Bus: BusObject  SampleTime=0  OutputAfterFinalValue=Extrapolation  Unit=inherit  PreserveSignalName=on
  Simulink-PS Converter : nesl_utility/Simulink-PS Converter  PhysicalDomain=network_engine_domain  SubClassName=ps_input  LeftPortType=input  RightPortType=output  PseudoPeriodic=off  Frequencies=[]  NoiseDistribution=none  NoiseParameters=[]  Unit=A  AffineConversion=off  FilteringAndDerivatives=zero  SimscapeFilterOrder=1  InputFilterTimeConstant=.001  UdotUserProvided=1
      settings: SourceProductBaseCode=PW,SS
  Simulink-PS Converter1 : nesl_utility/Simulink-PS Converter  PhysicalDomain=network_engine_domain  SubClassName=ps_input  LeftPortType=input  RightPortType=output  PseudoPeriodic=off  Frequencies=[]  NoiseDistribution=none  NoiseParameters=[]  Unit=degC  AffineConversion=on  FilteringAndDerivatives=zero  SimscapeFilterOrder=1  InputFilterTimeConstant=.001  UdotUserProvided=1
      settings: SourceProductBaseCode=PW,SS
  Simulink-PS Converter2 : nesl_utility/Simulink-PS Converter  PhysicalDomain=network_engine_domain  SubClassName=ps_input  LeftPortType=input  RightPortType=output  PseudoPeriodic=off  Frequencies=[]  NoiseDistribution=none  NoiseParameters=[]  Unit=A  AffineConversion=off  FilteringAndDerivatives=zero  SimscapeFilterOrder=1  InputFilterTimeConstant=.001  UdotUserProvided=0
      settings: SourceProductBaseCode=PW,SS
  Solver Configuration : nesl_utility/Solver Configuration  PhysicalDomain=network_engine_domain  SubClassName=solver  LeftPortType=input  RightPortType=generic  Tones=[]  Harmonics=[]  SimulateNoise=off  Profile=off  UseLocalSampling=off  EnableSwitchedLinearOptims=on  FrequencyDomain=off  UseCCode=off  RelTol=0.001  AbsTol=1e-06  MinStep=1e-09  ToWorkspace=off  RevertToSquareIcSolve=off  NumHomotopyIterations=100  PhasorMode=off  PhasorModeNumHarmonics=1  DoDC=off  ResidualTolerance=1e-9  UseLocalSolver=off  LocalSolverChoice=NE_BACKWARD_EULER_ADVANCER  LocalSolverSampleTime=1  DoFixedCost=off  MaxNonlinIter=3  MaxModeIter=2  ComputeImpulses=off  ImpulseIterations=2  LinearAlgebra=Sparse  EquationFormulation=NE_TIME_EF  DelaysMemoryBudget=1024  AutomaticFiltering=on  FilteringTimeConstant=0.001  PartitionStorageMethod=AS_NEEDED  PartitionMemoryBudget=1024  PartitionMethod=FAST
      settings: SourceProductBaseCode=PW,SS
  Solver Configuration1 : nesl_utility/Solver Configuration  PhysicalDomain=network_engine_domain  SubClassName=solver  LeftPortType=input  RightPortType=generic  Tones=[]  Harmonics=[]  SimulateNoise=off  Profile=off  UseLocalSampling=off  EnableSwitchedLinearOptims=on  FrequencyDomain=off  UseCCode=off  RelTol=0.001  AbsTol=1e-06  MinStep=1e-09  ToWorkspace=off  RevertToSquareIcSolve=off  NumHomotopyIterations=100  PhasorMode=off  PhasorModeNumHarmonics=1  DoDC=off  ResidualTolerance=1e-9  UseLocalSolver=off  LocalSolverChoice=NE_BACKWARD_EULER_ADVANCER  LocalSolverSampleTime=.001  DoFixedCost=off  MaxNonlinIter=12  MaxModeIter=2  ComputeImpulses=off  ImpulseIterations=2  LinearAlgebra=Sparse  EquationFormulation=NE_TIME_EF  DelaysMemoryBudget=1024  AutomaticFiltering=on  FilteringTimeConstant=0.001  PartitionStorageMethod=AS_NEEDED  PartitionMemoryBudget=1024  PartitionMethod=FAST
      settings: SourceProductBaseCode=PW,SS
  Subsystem : Subsystem
  Subsystem1 : Subsystem
  Temperature Sensor : fl_lib/Thermal/Thermal Sensors/Temperature Sensor
  Terminator : Terminator
  Terminator1 : Terminator
  Thermal Reference : fl_lib/Thermal/Thermal Elements/Thermal Reference
  Thermal Reference1 : fl_lib/Thermal/Thermal Elements/Thermal Reference
  Voltage : nesl_utility/PS-Simulink Converter  PhysicalDomain=network_engine_domain  SubClassName=ps_output  LeftPortType=input  RightPortType=output  PseudoPeriodic=off  Frequencies=[]  Unit=1  AffineConversion=off
      settings: SourceProductBaseCode=PW,SS
  Voltage sensor : Subsystem
  Voltage Sensor{,1..3} (4 alike) : fl_lib/Electrical/Electrical Sensors/Voltage Sensor
  convection : fl_lib/Thermal/Thermal Elements/Convective Heat Transfer  area=Battery.cell_area m^2  heat_tr_coeff=Battery.h_conv W/(m^2*K)  T_specify=off  T_priority=None  T=0 K  T_nominal_specify=off  T_nominal_unit=K  T_nominal_value=1  Q_specify=off  Q_priority=None  Q=0 J/s  Q_nominal_specify=off  Q_nominal_unit=J/s  Q_nominal_value=1
  "current " : nesl_utility/PS-Simulink Converter  PhysicalDomain=network_engine_domain  SubClassName=ps_output  LeftPortType=input  RightPortType=output  PseudoPeriodic=off  Frequencies=[]  Unit=1  AffineConversion=off
      settings: SourceProductBaseCode=PW,SS
  powergui : spspowerguiLib/powergui  Priority=1  SimulationMode=Discrete  SampleTime=1  frequency=60  Iterations=50  frequencyindice=0  Pbase=100e6  ErrMax=1e-4  UnitsV=kV  UnitsW=MW  buscounter=0  FunctionMessages=off  echomessages=off  EnableUseOfTLC=off  CurrentSourceSwitches=off  DisableSnubberDevices=off  DisableRonSwitches=off  DisableVfSwitches=off  DisplayEquations=off  AutomaticDiscreteSolvers=off  SolverType=Tustin/Backward Euler (TBE)  Interpol=off  ExternalGateDelay=off  methode=off  Ts=100  x0status=blocks  SPID=off  SwTol=0  HookPort=off  NonlinearTolerance=1e-4  nMaxIteration=100  ContinueOnMaxIteration=off  RestoreLinks=warning  ResistiveCurrentMeasurement=off  Frange=[0:2:500]  Ylog=off  Xlog=on  ShowGrid=off  save=off  variable=ZData  structure=0  ZoomFFT=off  StartTime=0.0  cycles=1  DisplayStyle=1  fundamental=60  FreqAxis=off  MaxFrequency=1000  frequencyindicesteady=1  RmsSteady=1  display=off
  powergui1 : spspowerguiLib/powergui  Priority=1  SimulationMode=Continuous  SampleTime=50e-6  frequency=60  Iterations=50  frequencyindice=0  Pbase=100e6  ErrMax=1e-4  UnitsV=kV  UnitsW=MW  buscounter=0  FunctionMessages=off  echomessages=off  EnableUseOfTLC=off  CurrentSourceSwitches=off  DisableSnubberDevices=off  DisableRonSwitches=off  DisableVfSwitches=off  DisplayEquations=off  AutomaticDiscreteSolvers=off  SolverType=Tustin/Backward Euler (TBE)  Interpol=off  ExternalGateDelay=off  methode=off  Ts=100  x0status=blocks  SPID=on  SwTol=0  HookPort=off  NonlinearTolerance=1e-4  nMaxIteration=100  ContinueOnMaxIteration=off  RestoreLinks=warning  ResistiveCurrentMeasurement=off  Frange=[0:2:500]  Ylog=off  Xlog=on  ShowGrid=off  save=off  variable=ZData  structure=0  ZoomFFT=off  StartTime=0.0  cycles=1  DisplayStyle=1  fundamental=60  FreqAxis=off  MaxFrequency=1000  frequencyindicesteady=1  RmsSteady=1  display=off
  V_out : Outport  VectorParamsAs1DForOutWhenUnconnected=off
  Scope5 : Scope
  Scope6 : Scope
  tag scope: I_load=global, temp=global
  wires:
  Lithium-Ion Battery/1 -> Lithium Battery Charger/1(Battery (m))
  Charging Current (A)/1 -> Lithium Battery Charger/2(Charge Current)
  MATLAB Function/2(g2) -> [g2]
  Bus Selector2/1 -> [SOC3], Display2/1  "<SOC (%)>"
  [g3] -> Product1/2
  MATLAB Function/1(g1) -> [g1]
  Constant1/1 -> Ideal Switch1/1
  Bus Selector1/1 -> [SOC2], Display1/1  "<SOC (%)>"
  Product2/1 -> IGBT2/1
  Constant2/1 -> Product1/1, Product/1, Product2/1
  Battery/1 -> Bus Selector/1
  [g1] -> Product2/2
  Constant/1 -> Ideal Switch/1
  [SOC1] -> MATLAB Function/1(u1)
  Battery1/1 -> Bus Selector1/1
  [SOC2] -> Scope3/2
  [SOC2] -> MATLAB Function/2(u2)
  [g2] -> Product/2
  Product1/1 -> IGBT/1
  Battery2/1 -> Bus Selector2/1
  [SOC1] -> Scope3/1
  Product/1 -> IGBT1/1
  [SOC3] -> Scope3/3
  MATLAB Function/3(g3) -> [g3]
  Bus Selector/1 -> [SOC1], Display/1  "<SOC (%)>"
  [SOC3] -> MATLAB Function/3(u3)
  Signal Builder/1 -> [I_load]
  Signal Builder/2 -> Simulink-PS Converter1/1
  [I_load] -> Simulink-PS Converter/1
  PS-Simulink Converter3/1 -> [temp], [T]
  [T] -> Scope4/4  "Temperature (degrees C)"
  [SOC] -> Scope4/3  "State of charge (SOC)"
  [V_load] -> Scope4/2  "Terminal voltage (V)"
  PS-Simulink Converter2/1 -> [SOC]
  [I_load] -> Scope4/1  "Charging/load current (A)"
  Current/1 -> Gain/1, Simulink-PS Converter2/1  "I_in"
  PS-Simulink Converter4/1 -> V_out/1  "V_Estimated"
  PS-Simulink Converter5/1 -> Terminator1/1  "SoC"
  Voltage1/1 -> Terminator/1  "V_Measured"
  [TCell10] -> Mux/1  "Cell 10"
  Voltage/1 -> Scope/1
  PS-Simulink Converter1/1 -> Scope2/1
  [TCell20] -> Mux/2  "Cell 20"
  PS-Simulink Converter/1 -> Scope1/1
  Mux/1 -> Cell temperatures/1
  "current "/1 -> Scope/2
  Divide/1 -> Discrete-Time Integrator/1
  Gain/1 -> Divide/1
  1-D Lookup Table/1 -> Divide/2  "Capacity"
  [temp] -> 1-D Lookup Table/1
  connections:
  Lithium-Ion Battery/LConn2 -- Lithium Battery Charger/RConn2
  Lithium Battery Charger/RConn1 -- Lithium-Ion Battery/LConn1
  Ideal Switch1/LConn1 -- Series RLC Branch2/LConn1 -- Ideal Switch/RConn1 -- Battery/LConn1
  IGBT1/RConn1 -- Battery1/LConn2 -- Series RLC Branch/LConn1 -- Battery2/LConn1
  IGBT2/RConn1 -- Battery/LConn2 -- Series RLC Branch1/LConn1 -- Battery1/LConn1
  Series RLC Branch3/RConn1 -- DC Voltage Source/LConn1 -- Battery2/LConn2 -- IGBT/RConn1
  Ideal Switch1/RConn1 -- Series RLC Branch3/LConn1
  IGBT2/LConn1 -- Series RLC Branch2/RConn1
  IGBT1/LConn1 -- Series RLC Branch1/RConn1
  DC Voltage Source/RConn1 -- Ideal Switch/LConn1
  IGBT/LConn1 -- Series RLC Branch/RConn1
  Solver Configuration/RConn1 -- Battery (Table-Based)/RConn1 -- Voltage sensor/RConn1 -- Input current/RConn2 -- Electrical Reference/LConn1
  Temperature Sensor/LConn1 -- Battery (Table-Based)/RConn2 -- convection/RConn1
  Battery (Table-Based)/LConn1 -- Voltage sensor/LConn1 -- Input current/LConn1
  Battery (Table-Based)/LConn2 -- PS-Simulink Converter2/LConn1
  Thermal Reference/LConn1 -- Ambient Temperature/RConn2
  Simulink-PS Converter1/RConn1 -- Ambient Temperature/RConn1
  Simulink-PS Converter/RConn1 -- Input current/RConn1
  PS-Simulink Converter3/LConn1 -- Temperature Sensor/RConn2
  Thermal Reference1/LConn1 -- Temperature Sensor/RConn1
  Ambient Temperature/LConn1 -- convection/LConn1
  Voltage Sensor3/LConn1 -- Battery current/LConn1 -- Solver Configuration1/RConn1 -- Battery (Table-Based)1/LConn1
  Battery (Table-Based)1/RConn1 -- Voltage Sensor3/RConn2 -- Battery current/RConn2 -- Electrical Reference1/LConn1
  PS-Simulink Converter5/LConn1 -- Battery (Table-Based)1/LConn2
  Battery current/RConn1 -- Simulink-PS Converter2/RConn1
  PS-Simulink Converter4/LConn1 -- Voltage Sensor3/RConn1
  Cell 01 to 09/LConn1 -- Convection Ambient- Cell 01-09/RConn1 -- Conduction Cell 09-10/LConn1
  "ERef "/LConn1 -- Cell 11 to 20/RConn1 -- Cyclic Charge/ Discharge Profile/RConn1 -- Voltage Sensor/RConn2
  Cell 10 Fault/LConn1 -- Conduction Cell 09-10/RConn1 -- "Conduction Cell 10-11 "/LConn1 -- Convection Ambient- Cell 10/RConn1 -- Subsystem1/LConn1
  Convection Ambient- Cell 11-20/LConn1 -- Convection Ambient- Cell 10/LConn1 -- Convection Ambient- Cell 01-09/LConn1 -- Ambient/RConn1
  Cell 11 to 20/LConn1 -- Convection Ambient- Cell 11-20/RConn1 -- "Conduction Cell 10-11 "/RConn1 -- Subsystem/LConn1
  Voltage Sensor1/LConn1 -- Cell 01 to 09/RConn1 -- Cell 10 Fault/LConn2 -- Voltage Sensor2/RConn2
  Cell 01 to 09/LConn2 -- Current Sensor/RConn2 -- Voltage Sensor2/LConn1
  Cell 11 to 20/LConn2 -- Cell 10 Fault/RConn1 -- Voltage Sensor1/RConn2
  Voltage Sensor/LConn1 -- Cyclic Charge/ Discharge Profile/LConn1 -- Current Sensor/LConn1
  Current Sensor/RConn1 -- "current "/LConn1
  Voltage Sensor1/RConn1 -- PS-Simulink Converter/LConn1
  Voltage Sensor/RConn1 -- Voltage/LConn1
  PS-Simulink Converter1/LConn1 -- Voltage Sensor2/RConn1

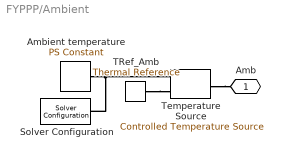
== system FYPPP/Ambient ==
  Ambient temperature : fl_lib/Physical Signals/Sources/PS Constant  constant=Battery.T_init
  Solver Configuration : nesl_utility/Solver Configuration  PhysicalDomain=network_engine_domain  SubClassName=solver  LeftPortType=input  RightPortType=generic  Tones=[]  Harmonics=[]  SimulateNoise=off  Profile=off  UseLocalSampling=off  EnableSwitchedLinearOptims=on  FrequencyDomain=off  UseCCode=off  RelTol=0.001  AbsTol=1e-06  MinStep=1e-09  ToWorkspace=off  RevertToSquareIcSolve=off  NumHomotopyIterations=100  PhasorMode=off  PhasorModeNumHarmonics=1  DoDC=off  ResidualTolerance=1e-9  UseLocalSolver=off  LocalSolverChoice=NE_BACKWARD_EULER_ADVANCER  LocalSolverSampleTime=1  DoFixedCost=off  MaxNonlinIter=3  MaxModeIter=2  ComputeImpulses=off  ImpulseIterations=2  LinearAlgebra=Sparse  EquationFormulation=NE_TIME_EF  DelaysMemoryBudget=1024  AutomaticFiltering=on  FilteringTimeConstant=0.001  PartitionStorageMethod=AS_NEEDED  PartitionMemoryBudget=1024  PartitionMethod=FAST
      settings: SourceProductBaseCode=PW,SS
  TRef_Amb : fl_lib/Thermal/Thermal Elements/Thermal Reference
  Temperature Source : fl_lib/Thermal/Thermal Sources/Controlled Temperature Source
  Amb : PMIOPort  Side=Right
  connections:
  TRef_Amb/LConn1 -- Temperature Source/RConn2
  Ambient temperature/RConn1 -- Solver Configuration/RConn1 -- Temperature Source/RConn1
  Temperature Source/LConn1 -- Amb/RConn1

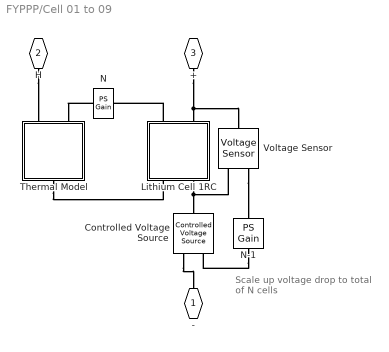
== system FYPPP/Cell 01 to 09 ==
  note: Scale up voltage drop
      | to total of N cells
  Controlled Voltage Source : fl_lib/Electrical/Electrical Sources/Controlled Voltage Source
  Lithium Cell 1RC : Subsystem  Tag=PublishSubsystem
      mask Display:
      | % Battery icon
      | plot([0 0 0.8 0.8],[0.2 0.9 0.9 1.5])
      | plot([0 0 0.8 0.8],-[0.2 0.9 0.9 1.5])
      | patch([-0.4 0.4 0.4 -0.4],[-0.45 -0.45 -0.15 -0.15],[0;0;0]);
      | patch([-0.9 0.9 0.9 -0.9],[0.15 0.15 0.45 0.45],[0;0;0]);
      | 
      | % Plot points to set plot range
      | color('white');plot(1.5,1.5);plot(-1.5,-1.5)
      | 
      | color('red')
      | port_label('RConn',1,'P')
      | port_label('RConn',2,'+')
      | port_label('LConn',1,'T')
      | port_label('LConn',2,'-')
  N : fl_ps_legacy_lib/Legacy Physical Signals/Functions/PS Gain  gain=Ncells
  N-1 : fl_ps_legacy_lib/Legacy Physical Signals/Functions/PS Gain  gain=(Ncells-1)
  Thermal Model : Subsystem
  Voltage Sensor : fl_lib/Electrical/Electrical Sensors/Voltage Sensor
  - : PMIOPort  Tag=PMCPort  Side=Right
  H : PMIOPort  Tag=PMCPort  Port=2  Side=Left
  + : PMIOPort  Tag=PMCPort  Port=3  Side=Left
  connections:
  Controlled Voltage Source/RConn2 -- -/RConn1
  N-1/RConn1 -- Controlled Voltage Source/RConn1
  +/RConn1 -- Voltage Sensor/LConn1 -- Lithium Cell 1RC/RConn2
  Voltage Sensor/RConn1 -- N-1/LConn1
  Lithium Cell 1RC/LConn2 -- Voltage Sensor/RConn2 -- Controlled Voltage Source/LConn1
  H/RConn1 -- Thermal Model/LConn1
  Thermal Model/RConn1 -- Lithium Cell 1RC/LConn1
  Lithium Cell 1RC/RConn1 -- N/LConn1
  N/RConn1 -- Thermal Model/LConn2

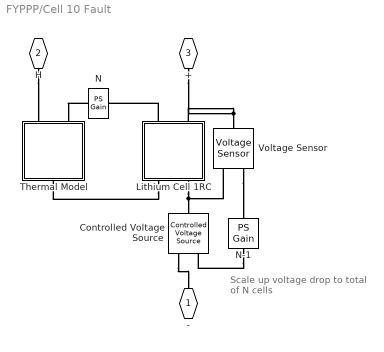
== system FYPPP/Cell 10 Fault ==
  note: Scale up voltage drop
      | to total of N cells
  Controlled Voltage Source : fl_lib/Electrical/Electrical Sources/Controlled Voltage Source
  Lithium Cell 1RC : Subsystem
      mask Display:
      | % Battery icon
      | plot([0 0 0.8 0.8],[0.2 0.9 0.9 1.5])
      | plot([0 0 0.8 0.8],-[0.2 0.9 0.9 1.5])
      | patch([-0.4 0.4 0.4 -0.4],[-0.45 -0.45 -0.15 -0.15],[0;0;0]);
      | patch([-0.9 0.9 0.9 -0.9],[0.15 0.15 0.45 0.45],[0;0;0]);
      | 
      | % Plot points to set plot range
      | color('white');plot(1.5,1.5);plot(-1.5,-1.5)
      | 
      | color('red')
      | port_label('RConn',1,'P')
      | port_label('RConn',2,'+')
      | port_label('LConn',1,'T')
      | port_label('LConn',2,'-')
  N : fl_ps_legacy_lib/Legacy Physical Signals/Functions/PS Gain  gain=Ncells
  N-1 : fl_ps_legacy_lib/Legacy Physical Signals/Functions/PS Gain  gain=(Ncells-1)
  Thermal Model : Subsystem
  Voltage Sensor : fl_lib/Electrical/Electrical Sensors/Voltage Sensor
  - : PMIOPort  Tag=PMCPort  Side=Right
  H : PMIOPort  Tag=PMCPort  Port=2  Side=Left
  + : PMIOPort  Tag=PMCPort  Port=3  Side=Left
  connections:
  Voltage Sensor/LConn1 -- Lithium Cell 1RC/RConn2 -- +/RConn1
  Controlled Voltage Source/LConn1 -- Lithium Cell 1RC/LConn2 -- Voltage Sensor/RConn2
  N/RConn1 -- Thermal Model/LConn2
  Lithium Cell 1RC/LConn1 -- Thermal Model/RConn1
  Controlled Voltage Source/RConn2 -- -/RConn1
  Voltage Sensor/RConn1 -- N-1/LConn1
  H/RConn1 -- Thermal Model/LConn1
  N-1/RConn1 -- Controlled Voltage Source/RConn1
  Lithium Cell 1RC/RConn1 -- N/LConn1

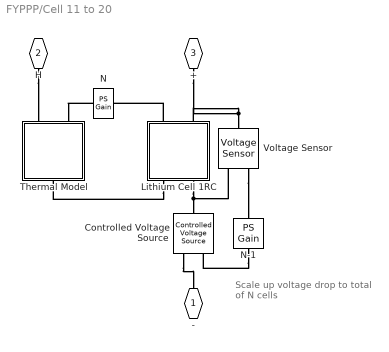
== system FYPPP/Cell 11 to 20 ==
  note: Scale up voltage drop
      | to total of N cells
  Controlled Voltage Source : fl_lib/Electrical/Electrical Sources/Controlled Voltage Source
  Lithium Cell 1RC : Subsystem
      mask Display:
      | % Battery icon
      | plot([0 0 0.8 0.8],[0.2 0.9 0.9 1.5])
      | plot([0 0 0.8 0.8],-[0.2 0.9 0.9 1.5])
      | patch([-0.4 0.4 0.4 -0.4],[-0.45 -0.45 -0.15 -0.15],[0;0;0]);
      | patch([-0.9 0.9 0.9 -0.9],[0.15 0.15 0.45 0.45],[0;0;0]);
      | 
      | % Plot points to set plot range
      | color('white');plot(1.5,1.5);plot(-1.5,-1.5)
      | 
      | color('red')
      | port_label('RConn',1,'P')
      | port_label('RConn',2,'+')
      | port_label('LConn',1,'T')
      | port_label('LConn',2,'-')
  N : fl_ps_legacy_lib/Legacy Physical Signals/Functions/PS Gain  gain=Ncells
  N-1 : fl_ps_legacy_lib/Legacy Physical Signals/Functions/PS Gain  gain=(Ncells-1)
  Thermal Model : Subsystem
  Voltage Sensor : fl_lib/Electrical/Electrical Sensors/Voltage Sensor
  - : PMIOPort  Tag=PMCPort  Side=Right
  H : PMIOPort  Tag=PMCPort  Port=2  Side=Left
  + : PMIOPort  Tag=PMCPort  Port=3  Side=Left
  connections:
  Voltage Sensor/LConn1 -- Lithium Cell 1RC/RConn2 -- +/RConn1
  Controlled Voltage Source/LConn1 -- Lithium Cell 1RC/LConn2 -- Voltage Sensor/RConn2
  Lithium Cell 1RC/RConn1 -- N/LConn1
  H/RConn1 -- Thermal Model/LConn1
  Controlled Voltage Source/RConn2 -- -/RConn1
  Voltage Sensor/RConn1 -- N-1/LConn1
  N-1/RConn1 -- Controlled Voltage Source/RConn1
  Lithium Cell 1RC/LConn1 -- Thermal Model/RConn1
  N/RConn1 -- Thermal Model/LConn2

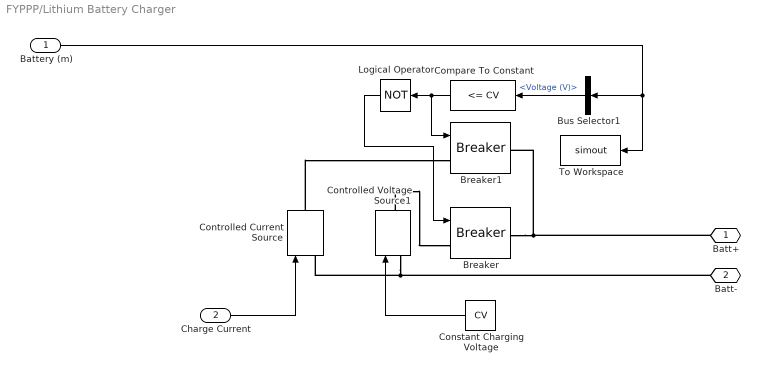
== system FYPPP/Lithium Battery Charger ==
  Battery (m) : Inport
  Charge Current : Inport  Port=2
  Breaker : spsBreakerLib/Breaker  InitialState=0  SwitchingTimes="[1/60  5/60]"  External=on  BreakerResistance=0.01  SnubberResistance=10e6  SnubberCapacitance=inf  Measurements=None  MoreParameters=on  NoBreakLoop=off
      settings: SourceProductBaseCode=PS
  Breaker1 : spsBreakerLib/Breaker  InitialState=0  SwitchingTimes="[1/60  5/60]"  External=on  BreakerResistance=0.01  SnubberResistance=1e6  SnubberCapacitance=inf  Measurements=None  MoreParameters=on  NoBreakLoop=off
      settings: SourceProductBaseCode=PS
  Bus Selector1 : BusSelector  OutputSignals=Voltage (V)
  Compare To Constant : simulink/Logic and Bit Operations/Compare To Constant  relop=<=  const=CV  OutDataTypeStr=boolean
  Constant Charging Voltage : Constant  Value=CV
  Controlled Current Source : spsControlledCurrentSourceLib/Controlled Current Source  Initialize=on  Source_Type=DC  Amplitude=0  Phase=0  Frequency=0  Measurements=None
  Controlled Voltage Source1 : spsControlledVoltageSourceLib/Controlled Voltage Source  Initialize=on  Source_Type=DC  Amplitude=0  Phase=0  Frequency=0  Measurements=None
  Logical Operator : Logic  Operator=NOT  AllPortsSameDT=off  OutDataTypeStr=boolean
  To Workspace : ToWorkspace  VariableName=simout  SampleTime=-1
  Batt+ : PMIOPort  Side=Right
  Batt- : PMIOPort  Port=2  Side=Right
  wires:
  Bus Selector1/1 -> Compare To Constant/1  "<Voltage (V)>"
  Constant Charging Voltage/1 -> Controlled Voltage Source1/1
  Battery (m)/1 -> To Workspace/1, Bus Selector1/1
  Logical Operator/1 -> Breaker/1
  Compare To Constant/1 -> Logical Operator/1, Breaker1/1
  Charge Current/1 -> Controlled Current Source/1
  connections:
  Breaker/RConn1 -- Batt+/RConn1 -- Breaker1/RConn1
  Controlled Voltage Source1/RConn1 -- Breaker/LConn1
  Controlled Current Source/RConn1 -- Breaker1/LConn1
  Controlled Voltage Source1/LConn1 -- Batt-/RConn1 -- Controlled Current Source/LConn1

== system FYPPP/Open GUI ==

== system FYPPP/Subsystem ==
  Ideal Temperature Sensor : fl_lib/Thermal/Thermal Sensors/Temperature Sensor
  PS-Simulink Converter1 : nesl_utility/PS-Simulink Converter  PhysicalDomain=network_engine_domain  SubClassName=ps_output  LeftPortType=input  RightPortType=output  PseudoPeriodic=off  Frequencies=[]  Unit=1  AffineConversion=off
      settings: SourceProductBaseCode=PW,SS
  Thermal Reference2 : fl_lib/Thermal/Thermal Elements/Thermal Reference
  T : PMIOPort  Side=Left
  tag scope: TCell20=global
  wires:
  PS-Simulink Converter1/1 -> [TCell20]
  connections:
  Thermal Reference2/LConn1 -- Ideal Temperature Sensor/RConn1
  Ideal Temperature Sensor/RConn2 -- PS-Simulink Converter1/LConn1
  Ideal Temperature Sensor/LConn1 -- T/RConn1

== system FYPPP/Subsystem1 ==
  Ideal Temperature Sensor : fl_lib/Thermal/Thermal Sensors/Temperature Sensor
  PS-Simulink Converter1 : nesl_utility/PS-Simulink Converter  PhysicalDomain=network_engine_domain  SubClassName=ps_output  LeftPortType=input  RightPortType=output  PseudoPeriodic=off  Frequencies=[]  Unit=1  AffineConversion=off
      settings: SourceProductBaseCode=PW,SS
  Thermal Reference2 : fl_lib/Thermal/Thermal Elements/Thermal Reference
  T : PMIOPort  Side=Left
  tag scope: TCell10=global
  wires:
  PS-Simulink Converter1/1 -> [TCell10]
  connections:
  Ideal Temperature Sensor/LConn1 -- T/RConn1
  Ideal Temperature Sensor/RConn2 -- PS-Simulink Converter1/LConn1
  Thermal Reference2/LConn1 -- Ideal Temperature Sensor/RConn1

== system FYPPP/Voltage sensor ==
  PS-Simulink Converter : nesl_utility/PS-Simulink Converter  PhysicalDomain=network_engine_domain  SubClassName=ps_output  LeftPortType=input  RightPortType=output  PseudoPeriodic=off  Frequencies=[]  Unit=V  AffineConversion=off
      settings: SourceProductBaseCode=PW,SS
  Voltage Sensor : fl_lib/Electrical/Electrical Sensors/Voltage Sensor
  + : PMIOPort  Side=Left
  - : PMIOPort  Port=2  Side=Right
  tag scope: V_load=global
  wires:
  PS-Simulink Converter/1 -> [V_load]
  connections:
  Voltage Sensor/RConn1 -- PS-Simulink Converter/LConn1
  +/RConn1 -- Voltage Sensor/LConn1
  -/RConn1 -- Voltage Sensor/RConn2
